simulink subsystem "CombineOuterLoopFB_with_FF_att_ref"  (R2023a)
settings: Solver=VariableStepAuto  StartTime=0.0  StopTime=10.0  RelTol=1e-3
libraries: aerolibutil x2, sharedtransform x2
settings Model: Creator=thesa  LastModifiedBy=thesa

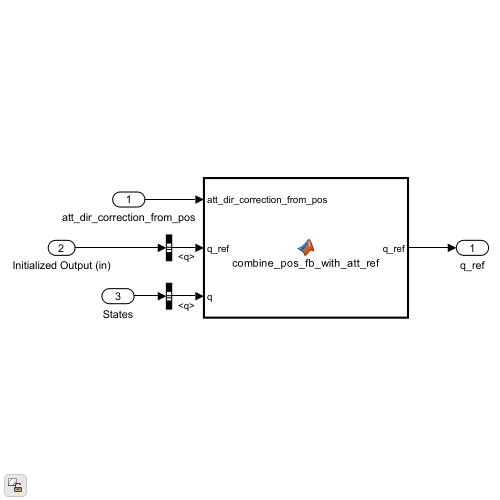
[thumbnail: Simulink's stored preview of the top-level diagram]
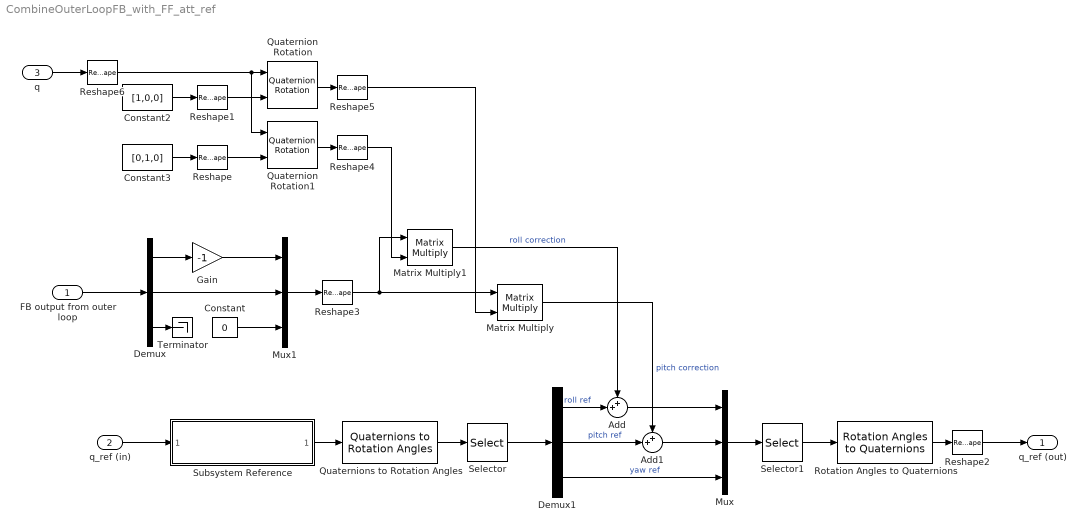
== system CombineOuterLoopFB_with_FF_att_ref ==
  FB output from outer loop : Inport
  q_ref (in) : Inport  Port=2
  q : Inport  Port=3
  Add : Sum  Inputs=++|
  Add1 : Sum  Inputs=++|
  Constant : Constant  Value=0
  Constant2 : Constant  Value=[1,0,0]
  Constant3 : Constant  Value=[0,1,0]
  Demux : Demux  Outputs=3
  Demux1 : Demux  Outputs=3
  Gain : Gain  Gain=-1
  Matrix Multiply : Product  Multiplication=Matrix(*)
  Matrix Multiply1 : Product  Multiplication=Matrix(*)
  Mux : Mux  Inputs=3
  Mux1 : Mux  Inputs=3
  Quaternion Rotation : aerolibutil/Quaternion Rotation
  Quaternion Rotation1 : aerolibutil/Quaternion Rotation
  Quaternions to Rotation Angles : sharedtransform/Quaternions to Rotation Angles  rotationOrder=ZYX  aMode=aMode
  Reshape{,1,4..5} (4 alike) : Reshape  OutputDimensionality=Column vector (2-D)
  Reshape2 : Reshape  OutputDimensionality=Row vector (2-D)
  Reshape3 : Reshape  OutputDimensionality=Row vector (2-D)
  Reshape6 : Reshape
  Rotation Angles to Quaternions : sharedtransform/Rotation Angles to Quaternions  rotationOrder=ZYX  aMode=aMode
  Selector : Selector  InputPortWidth=3  IndexOptions=Index vector (dialog)  Indices=[3 2 1]  OutputSizes=1
  Selector1 : Selector  InputPortWidth=3  IndexOptions=Index vector (dialog)  Indices=[3 2 1]  OutputSizes=1
  Subsystem Reference : Subsystem  ReferencedSubsystem=Check_Quat
  Terminator : Terminator
  q_ref (out) : Outport
  wires:
  Rotation Angles to Quaternions/1 -> Reshape2/1
  q_ref (in)/1 -> Subsystem Reference/1
  FB output from outer loop/1 -> Demux/1
  Demux/3 -> Terminator/1
  Constant/1 -> Mux1/3
  Demux/1 -> Gain/1
  Gain/1 -> Mux1/1
  Demux/2 -> Mux1/2
  q/1 -> Reshape6/1
  Constant2/1 -> Reshape1/1
  Constant3/1 -> Reshape/1
  Reshape/1 -> Quaternion Rotation1/2
  Reshape1/1 -> Quaternion Rotation/2
  Mux1/1 -> Reshape3/1
  Quaternion Rotation1/1 -> Reshape4/1
  Quaternion Rotation/1 -> Reshape5/1
  Reshape3/1 -> Matrix Multiply/1, Matrix Multiply1/1
  Reshape4/1 -> Matrix Multiply1/2
  Reshape5/1 -> Matrix Multiply/2
  Quaternions to Rotation Angles/1 -> Selector/1
  Selector/1 -> Demux1/1
  Demux1/1 -> Add/2  "roll ref"
  Demux1/2 -> Add1/2  "pitch ref"
  Matrix Multiply1/1 -> Add/1  "roll correction"
  Matrix Multiply/1 -> Add1/1  "pitch correction"
  Demux1/3 -> Mux/3  "yaw ref"
  Add1/1 -> Mux/2
  Add/1 -> Mux/1
  Mux/1 -> Selector1/1
  Selector1/1 -> Rotation Angles to Quaternions/1
  Reshape2/1 -> q_ref (out)/1
  Reshape6/1 -> Quaternion Rotation/1, Quaternion Rotation1/1
  Subsystem Reference/1 -> Quaternions to Rotation Angles/1
